simulink model "FSK"  (R2022b)
settings: Solver=VariableStepAuto  StartTime=0.0  StopTime=10.0  MaxStep=0.001  RelTol=1e-3
libraries: simulink x1, commsynccomp2 x1
settings Model: Creator=User  LastModifiedBy=User

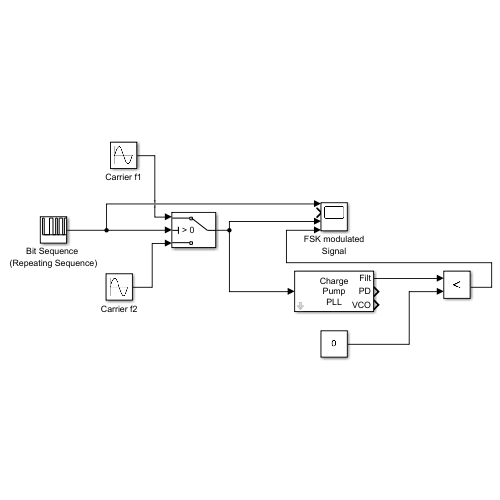
[thumbnail: Simulink's stored preview of the top-level diagram]
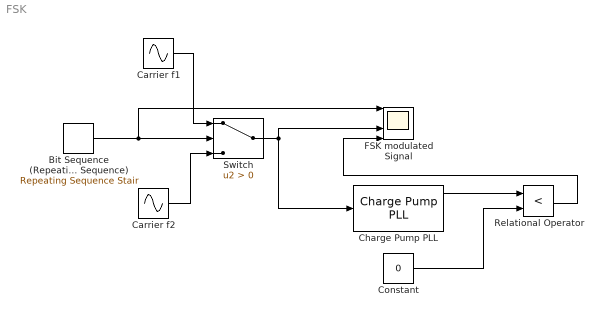
== system FSK ==
  Bit Sequence (Repeating Sequence) : simulink/Sources/Repeating Sequence Stair  OutValues=[1 0 0 0 1 1 0 0 1 0 1 1 0 1].'  tsamp=1  OutMin=[]  OutMax=[]  OutDataTypeStr=double  OutputDataTypeScalingMode=double  OutDataType=fixdt(0,8)  ConRadixGroup=Best Precision: Vector-wise  OutScaling=2^-12
  Carrier f1 : Sin  Frequency=2*pi*4  SampleTime=0
  Carrier f2 : Sin  Frequency=2*pi*2  SampleTime=0
  Charge Pump PLL : commsynccomp2/Charge Pump PLL  Fn=[2*pi*2]  Fd="[1   2*pi*2]"  Kvco=10  Fc=10  Ph=0  Ac=1
  Constant : Constant  Value=0
  FSK modulated Signal : Scope  NumInputPorts=4
  Relational Operator : RelationalOperator  Operator=<  OutDataTypeStr=boolean  RndMeth=Simplest  InputSameDT=off
  Switch : Switch  Criteria=u2 > Threshold  SaturateOnIntegerOverflow=off  InputSameDT=off
  wires:
  Bit Sequence (Repeating Sequence)/1 -> FSK modulated Signal/1, Switch/2
  Carrier f1/1 -> Switch/1
  Switch/1 -> FSK modulated Signal/3, Charge Pump PLL/1
  Carrier f2/1 -> Switch/3
  Charge Pump PLL/1 -> Relational Operator/1
  Constant/1 -> Relational Operator/2
  Relational Operator/1 -> FSK modulated Signal/4
